simulink model "CaseStudy_Simulink"  (R2019b)
settings: Solver=VariableStepAuto  StartTime=0.0  StopTime=950  RelTol=1e-3
model workspace (MAT data in the model file):
  Making_Order = Simulink.Parameter
  Making_Order.Value = 0
  Making_Order.DataType = 'auto'
  Making_Order.Dimensions = [1 1]
undefined symbols (not defined in the file or in its folder): Clculate_ProccessTime, entity, Faulty_Unit_Identification, genNewOrder, m, n, Packaging
settings Model: PacingRate=1.100000  OrderedModelArguments=off  Creator=faedaa  LastModifiedBy=faedaa

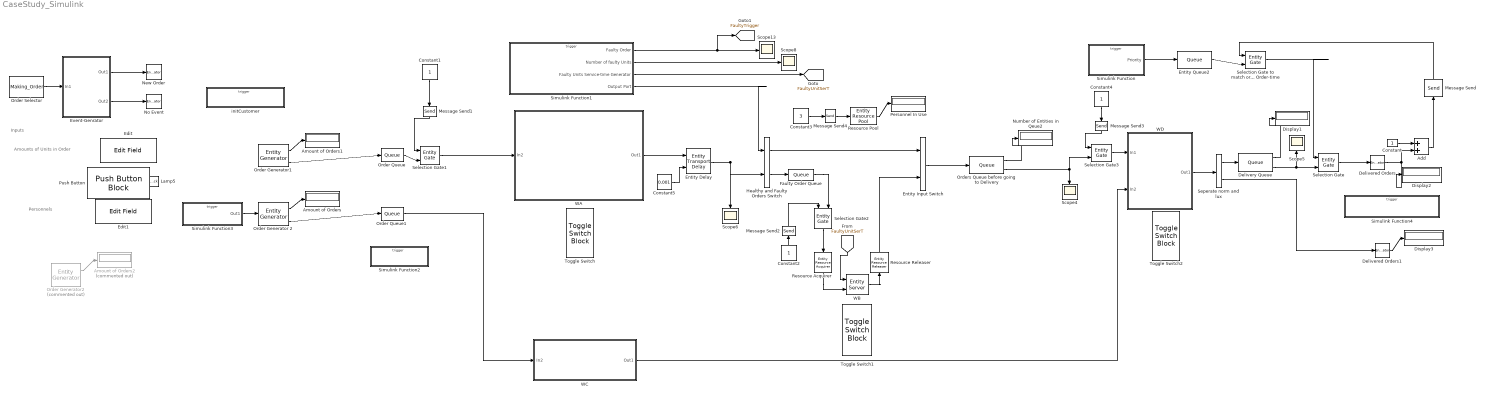
== system CaseStudy_Simulink ==
  note: Inputs
  note: Amounts of Units in Order
  note: Personnels
  Add : Sum  Inputs=2
  Amount of Orders : Display
  Amount of Orders1 : Display
  Amount of Orders2 : Display  Commented=on
  Constant{,1..2,4} (4 alike) : Constant
  Constant3 : Constant  Value=3
  Constant5 : Constant  Value=0.001
  Delivered Orders : EntityTerminator  InputPortMessageModes=m  EntryAction=Clculate_ProccessTime(entity.StartTime,entity.pr,entity.Tag_ManualOrders);  NumberEntitiesArrived=on
      settings: OutputPortMap=o0
  Delivered Orders1 : EntityTerminator  InputPortMessageModes=m  EntryAction=Clculate_ProccessTime(entity.StartTime,entity.pr,entity.Tag_ManualOrders);  NumberEntitiesArrived=on
      settings: OutputPortMap=o0
  Delivery Queue : Queue  InputPortMessageModes=m  OutputPortMessageModes=n,m  Capacity=inf  QueueType=Priority  PrioritySource=pr  NumberEntitiesInBlock=on
      settings: OutputPortMap=o1,o5
  Display1 : Display
  Display2 : Display
  Display3 : Display
  Edit : EditField  LabelPosition=Hide  ShowInitialText=on  Alignment=Center
  Edit1 : EditField  LabelPosition=Hide  ShowInitialText=on  Alignment=Center
  Entity Delay : EntityTransportDelay  InputPortMessageModes=m,n  OutputPortMessageModes=m  Capacity=1
  Entity Input Switch : EntityInputSwitch  InputPortMessageModes=m,m  OutputPortMessageModes=m
  Entity Queue2 : Queue  InputPortMessageModes=m  OutputPortMessageModes=m  Capacity=inf
  Event-Genrator : Subsystem
  Faulty Order Queue : Queue  InputPortMessageModes=m  OutputPortMessageModes=m  Capacity=inf
  Healthy and Faulty Orders Switch : EntityOutputSwitch  InputPortMessageModes=m,m  OutputPortMessageModes=m,m  SwitchingCriterion=From control port  SwitchAttributeName=Attribute1
      settings: InputPortMap=u0,u1
  Lamp5 : LampBlock  LabelPosition=Hide
  Message Send{,1..4} (5 alike) : Send  OutputPortMessageModes=m
  New Order : EntityTerminator  InputPortMessageModes=m  EntryAction=genNewOrder();
  No Event : EntityTerminator  InputPortMessageModes=m
  Number of Entities in Qeue2 : Display
  Order Generator 2 : EntityGenerator  InputPortMessageModes=m  OutputPortMessageModes=n,m  GenerationMethod=Event-based  TimeSource=MATLAB action  IntergenerationTimeAction=|  GenerateAction=entity.Units = Units_Assign();  AttributeName=Units|pr|StartTime|Tag_ManualOrders  AttributeInitialValue=1|0|0|2  NumberEntitiesDeparted=on  EntityType=Structured  EntityTypeName=Entity  DataInitialValue=Units_Amounts
      | persistent rngInit;
      | if isempty(rngInit)
      |     seed = 12345;
      |     rng(seed);
      |     rngInit = true;
      | end
      | 
      | % Pattern: Exponential distribution
      | mu = 30;
      | dt = -mu * log(1 - rand());
      settings: InputPortMap=u0  OutputPortMap=o0,o3
  Order Generator1 : EntityGenerator  OutputPortMessageModes=n,m  TimeSource=MATLAB action  Period=0  IntergenerationTimeAction=|  GenerateAction=|  AttributeName=Units|pr|StartTime|Tag_ManualOrders  AttributeInitialValue=1|0|0|1  NumberEntitiesDeparted=on  EntityType=Structured  EntityTypeName=Entity
      | persistent rngInit;
      | if isempty(rngInit)
      |     seed = 1;
      |     rng(seed);
      |     rngInit = true;
      | end
      | 
      | % Pattern: Exponential distribution
      | mu = 40;
      | dt = -mu * log(1 - rand());
      | persistent rngInit;
      | if isempty(rngInit)
      |     seed = 12345;
      |     rng(seed);
      |     rngInit = true;
      | end
      | 
      | % Pattern: Uniform distribution
      | % m: Minimum, M: Maximum
      | m = 5; M = 100;
      | entity.Units = round(m + (M - m) * rand);
      settings: OutputPortMap=o0,o3
  Order Generator2 : EntityGenerator  Commented=on  OutputPortMessageModes=n,m  TimeSource=MATLAB action  Period=0  IntergenerationTimeAction=|  GenerateEntityAtSimulationStart=off  GenerateAction=|  AttributeName=Units|pr|StartTime|Tag_ManualOrders  AttributeInitialValue=1|0|0|2  NumberEntitiesDeparted=on  EntityType=Structured  EntityTypeName=Entity
      | persistent rngInit;
      | if isempty(rngInit)
      |     seed = 154;
      |     rng(seed);
      |     rngInit = true;
      | end
      | 
      | % Pattern: Exponential distribution
      | mu = 200;
      | dt = -mu * log(1 - rand());
      | persistent rngInit;
      | if isempty(rngInit)
      |     seed = 111;
      |     rng(seed);
      |     rngInit = true;
      | end
      | 
      | % Pattern: Uniform distribution
      | % m: Minimum, M: Maximum
      | m = 1; M = 6;
      | entity.Units = round(m + (M - m) * rand);
      settings: OutputPortMap=o0,o3
  Order Queue : Queue  InputPortMessageModes=m  OutputPortMessageModes=m  Capacity=inf  EntryAction=|
      | persistent idx;
      | if isempty(idx)
      |     idx = 1;
      | end
      | entity.pr = idx
      | idx = idx + 1;
      | 
      | ControlInputpr(entity.pr);
      | 
      | 
      | t = getCurrentTime();
      | entity.StartTime = t/60;
  Order Queue1 : Queue  InputPortMessageModes=m  OutputPortMessageModes=m  Capacity=inf  EntryAction=|
      | persistent id;
      | if isempty(id)
      |     id = 1;
      | end
      | entity.pr = id
      | id = id + 1;
      | 
      | t = getCurrentTime();
      | entity.StartTime = t/60;
  Order Selector : Constant  Value=Making_Order
  Orders Queue before going to Delivery : Queue  InputPortMessageModes=m  OutputPortMessageModes=n,m  Capacity=inf  ExitAction=Packaging(entity.Units)  NumberEntitiesInBlock=on
      settings: OutputPortMap=o1,o5
  Personnel In Use : Display
  Push Button : PushButtonBlock  ButtonText=Make Order
  Resource Acquirer : EntityResourceAcquirer  InputPortMessageModes=m  OutputPortMessageModes=m  ResourceName=WorkerB
      settings: OutputPortMap=o3
  Resource Releaser : EntityResourceReleaser  InputPortMessageModes=m  OutputPortMessageModes=m  ResourceToRelease=Selected  ResourceName=WorkerB  ResourceAmount=1
  Resource Pool : EntityResourcePool  InputPortMessageModes=m  ResourceName=WorkerB  ResourceAmountSource=Change amount through control port  ResourceAmount=2  InitialResourceAmount=0  AmountInUse=on
  Scope{4..6,8,13} (5 alike) : Scope
  Selection Gate : EntityGate  InputPortMessageModes=m,m  OutputPortMessageModes=m  OperatingMode=Selection gate  MatchingAttributeName=pr
  Selection Gate to match orders based on Order-time : EntityGate  InputPortMessageModes=m,m  OutputPortMessageModes=m  OperatingMode=Selection gate  MatchingAttributeName=entity
  Selection Gate1 : EntityGate  InputPortMessageModes=m,m  OutputPortMessageModes=m  MatchingAttributeName=entity
  Selection Gate2 : EntityGate  InputPortMessageModes=m,m  OutputPortMessageModes=m  MatchingAttributeName=entity
  Selection Gate3 : EntityGate  InputPortMessageModes=m,m  OutputPortMessageModes=m  MatchingAttributeName=entity
  "Seperate norm and lux " : EntityOutputSwitch  InputPortMessageModes=m  OutputPortMessageModes=m,m  SwitchingCriterion=From attribute  SwitchAttributeName=Tag_ManualOrders
  Simulink Function : Subsystem  TreatAsAtomicUnit=on
  Simulink Function1 : Subsystem  TreatAsAtomicUnit=on
  Simulink Function2 : Subsystem  TreatAsAtomicUnit=on
  Simulink Function3 : Subsystem  TreatAsAtomicUnit=on
  Simulink Function4 : Subsystem  TreatAsAtomicUnit=on
  Toggle Switch : ToggleSwitchBlock  LabelPosition=Hide
      settings: Values={{'Off', 'On'}, [0 1]}
  Toggle Switch1 : ToggleSwitchBlock  LabelPosition=Hide
      settings: Values={{'Off', 'On'}, [0 1]}
  Toggle Switch2 : ToggleSwitchBlock  LabelPosition=Hide
      settings: Values={{'Off', 'On'}, [0 1]}
  WA : Subsystem
  WB : EntityServer  InputPortMessageModes=n,m  OutputPortMessageModes=m  Capacity=1  ServiceTimeSource=Signal port  ServiceTimeAction=|
      | persistent rngInit;
      | if isempty(rngInit)
      |     seed = 12345;
      |     rng(seed);
      |     rngInit = true;
      | end
      | 
      | % Pattern: Exponential distribution
      | mu = 20;
      | dt = -mu * log(1 - rand());
      settings: InputPortMap=u0,u2
  WC : Subsystem
  WD : Subsystem
  initCustomer : Subsystem  TreatAsAtomicUnit=on
  tag scope: FaultyTrigger=global, FaultyUnitSerT=global
  wires:
  Simulink Function/1(Priority) -> Entity Queue2/1
  Resource Releaser/1 -> Entity Input Switch/2
  Simulink Function1/4(Output Port) -> Healthy and Faulty Orders Switch/1
  Resource Acquirer/1 -> WB/2
  Simulink Function1/2(Number of faulty Units) -> Scope8/1
  Constant/1 -> Add/1
  Entity Queue2/1 -> Selection Gate to match orders based on Order-time/2
  Order Generator 2/1 -> Amount of Orders/1
  Event-Genrator/1(Out1) -> New Order/1
  Orders Queue before going to Delivery/1 -> Number of Entities in Qeue2/1
  Simulink Function1/3(Faulty Units Service-time Generator) -> [FaultyUnitSerT]
  WB/1 -> Resource Releaser/1
  Simulink Function3/1(Out1) -> Order Generator 2/1
  Event-Genrator/2(Out2) -> No Event/1
  Delivery Queue/1 -> Display1/1
  Healthy and Faulty Orders Switch/1 -> Entity Input Switch/1
  Delivery Queue/2 -> Selection Gate/2, Scope5/1
  Order Selector/1 -> Event-Genrator/1(In1)
  Message Send/1 -> Selection Gate to match orders based on Order-time/1
  [FaultyUnitSerT] -> WB/1
  Selection Gate to match orders based on Order-time/1 -> Selection Gate/1
  Add/1 -> Message Send/1
  Healthy and Faulty Orders Switch/2 -> Faulty Order Queue/1
  Delivered Orders/1 -> Add/2, Display2/1
  Simulink Function1/1(Faulty Order) -> Scope13/1, [FaultyTrigger]
  Order Generator1/1 -> Amount of Orders1/1
  Constant1/1 -> Message Send1/1
  Message Send1/1 -> Selection Gate1/1
  Selection Gate1/1 -> WA/1(In2)
  Faulty Order Queue/1 -> Selection Gate2/2
  Selection Gate2/1 -> Resource Acquirer/1
  Constant2/1 -> Message Send2/1
  Message Send2/1 -> Selection Gate2/1
  Constant4/1 -> Message Send3/1
  Message Send3/1 -> Selection Gate3/1
  Orders Queue before going to Delivery/2 -> Selection Gate3/2, Scope4/1
  Selection Gate3/1 -> WD/1(In1)
  Constant3/1 -> Message Send4/1
  Message Send4/1 -> Resource Pool/1
  Resource Pool/1 -> Personnel In Use/1
  Constant5/1 -> Entity Delay/2
  WA/1(Out1) -> Entity Delay/1
  Entity Delay/1 -> Scope6/1, Healthy and Faulty Orders Switch/2
  Order Generator1/2 -> Order Queue/1
  WC/1(Out1) -> WD/2(In2)
  Entity Input Switch/1 -> Orders Queue before going to Delivery/1
  Order Queue/1 -> Selection Gate1/2
  Order Queue1/1 -> WC/1(In2)
  WD/1(Out1) -> "Seperate norm and lux "/1
  "Seperate norm and lux "/1 -> Delivery Queue/1
  "Seperate norm and lux "/2 -> Delivered Orders1/1
  Delivered Orders1/1 -> Display3/1
  Selection Gate/1 -> Delivered Orders/1
  Order Generator2/1 -> Amount of Orders2/1
  Order Generator 2/2 -> Order Queue1/1

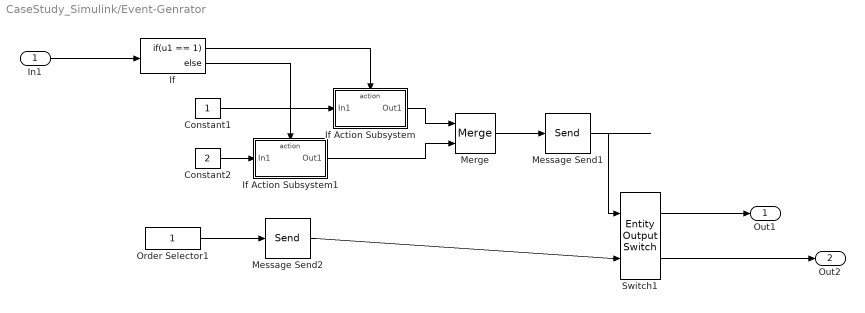
== system CaseStudy_Simulink/Event-Genrator ==
  In1 : Inport
  Constant1 : Constant
  Constant2 : Constant  Value=2
  If : If  IfExpression=u1 == 1
  If Action Subsystem : Subsystem  TreatAsAtomicUnit=on
  If Action Subsystem1 : Subsystem  TreatAsAtomicUnit=on
  Merge : Merge
  Message Send1 : Send  OutputPortMessageModes=m
  Message Send2 : Send  OutputPortMessageModes=m
  Order Selector1 : Constant
  Switch1 : EntityOutputSwitch  InputPortMessageModes=m,m  OutputPortMessageModes=m,m  SwitchingCriterion=From control port  SwitchAttributeName=Attribute1  InitialPortSelection=2
      settings: InputPortMap=u0,u1
  Out1 : Outport
  Out2 : Outport  Port=2
  wires:
  If Action Subsystem/1(Out1) -> Merge/1
  Message Send1/1 -> Switch1/1
  Switch1/2 -> Out2/1
  Constant2/1 -> If Action Subsystem1/1(In1)
  Constant1/1 -> If Action Subsystem/1(In1)
  If/2 -> If Action Subsystem1/Action
  If/1 -> If Action Subsystem/Action
  Message Send2/1 -> Switch1/2
  If Action Subsystem1/1(Out1) -> Merge/2
  Order Selector1/1 -> Message Send2/1
  Merge/1 -> Message Send1/1
  In1/1 -> If/1
  Switch1/1 -> Out1/1

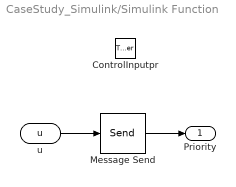
== system CaseStudy_Simulink/Simulink Function ==
  ControlInputpr : TriggerPort  TriggerType=function-call  IsSimulinkFunction=on  FunctionName=ControlInputpr  VariantControl=(inherit)
  Message Send : Send  OutputPortMessageModes=m
  u : ArgIn  DisableCoverage=on  ArgumentName=u
  Priority : Outport
  wires:
  Message Send/1 -> Priority/1
  u/1 -> Message Send/1

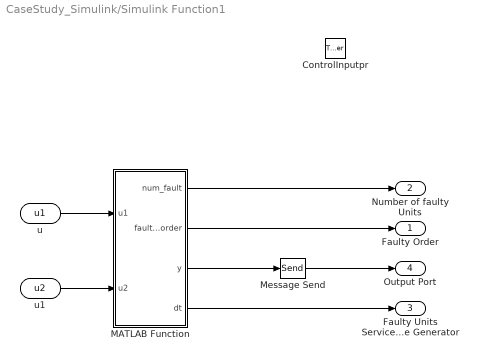
== system CaseStudy_Simulink/Simulink Function1 ==
  ControlInputpr : TriggerPort  TriggerType=function-call  IsSimulinkFunction=on  FunctionName=Faulty_Unit_Identification  VariantControl=(inherit)
  MATLAB Function : MATLAB Function  TreatAsAtomicUnit=on
  Message Send : Send  OutputPortMessageModes=m
  u : ArgIn  DisableCoverage=on  ArgumentName=u1
  u1 : ArgIn  DisableCoverage=on  Port=2  ArgumentName=u2
  Faulty Order : Outport
  Number of faulty Units : Outport  Port=2
  Faulty Units Service-time Generator : Outport  Port=3
  Output Port : Outport  Port=4
  wires:
  Message Send/1 -> Output Port/1
  u/1 -> MATLAB Function/1(u1)
  MATLAB Function/3(y) -> Message Send/1
  MATLAB Function/4(dt) -> Faulty Units Service-time Generator/1
  u1/1 -> MATLAB Function/2(u2)
  MATLAB Function/1(num_fault) -> Number of faulty Units/1
  MATLAB Function/2(faulty_order) -> Faulty Order/1

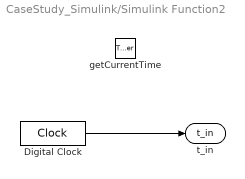
== system CaseStudy_Simulink/Simulink Function2 ==
  getCurrentTime : TriggerPort  TriggerType=function-call  IsSimulinkFunction=on  FunctionName=getCurrentTime  VariantControl=Variant
  Digital Clock : DigitalClock  SampleTime=-1
  t_in : ArgOut  DisableCoverage=on  ArgumentName=t_in
  wires:
  Digital Clock/1 -> t_in/1

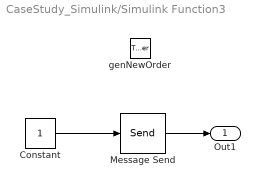
== system CaseStudy_Simulink/Simulink Function3 ==
  genNewOrder : TriggerPort  TriggerType=function-call  IsSimulinkFunction=on  FunctionName=genNewOrder  VariantControl=Variant
  Constant : Constant
  Message Send : Send  OutputPortMessageModes=m
  Out1 : Outport  VectorParamsAs1DForOutWhenUnconnected=off
  wires:
  Constant/1 -> Message Send/1
  Message Send/1 -> Out1/1

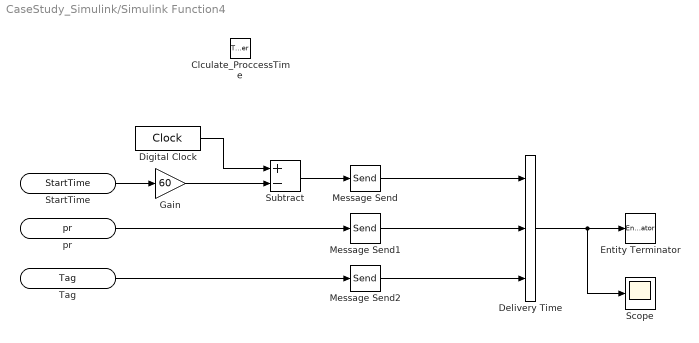
== system CaseStudy_Simulink/Simulink Function4 ==
  Clculate_ProccessTime : TriggerPort  TriggerType=function-call  IsSimulinkFunction=on  FunctionName=Clculate_ProccessTime  VariantControl=Variant
  "Delivery Time " : EntityInputSwitch  InputPortMessageModes=m,m,m  OutputPortMessageModes=m  NumberInputPorts=3
      settings: InputPortMap=u1,u2,u3
  Digital Clock : DigitalClock  SampleTime=-1
  Entity Terminator : EntityTerminator  InputPortMessageModes=m
  Gain : Gain  Gain=60
  Message Send : Send  OutputPortMessageModes=m
  Message Send1 : Send  OutputPortMessageModes=m
  Message Send2 : Send  OutputPortMessageModes=m
  Scope : Scope
  Subtract : Sum  Inputs=+-
  StartTime : ArgIn  DisableCoverage=on  ArgumentName=StartTime
  pr : ArgIn  DisableCoverage=on  Port=2  ArgumentName=pr
  Tag : ArgIn  DisableCoverage=on  Port=3  ArgumentName=Tag
  wires:
  StartTime/1 -> Gain/1
  Digital Clock/1 -> Subtract/1
  Subtract/1 -> Message Send/1
  pr/1 -> Message Send1/1
  "Delivery Time "/1 -> Scope/1, Entity Terminator/1
  Message Send/1 -> "Delivery Time "/1
  Message Send1/1 -> "Delivery Time "/2
  Gain/1 -> Subtract/2
  Tag/1 -> Message Send2/1
  Message Send2/1 -> "Delivery Time "/3

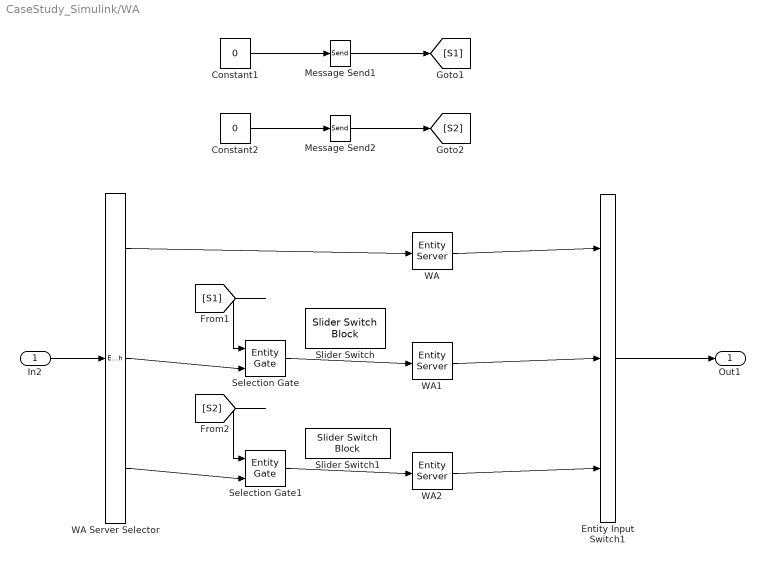
== system CaseStudy_Simulink/WA ==
  In2 : Inport
  Constant1 : Constant  Value=0
  Constant2 : Constant  Value=0
  Entity Input Switch1 : EntityInputSwitch  InputPortMessageModes=m,m,m  OutputPortMessageModes=m  NumberInputPorts=3
      settings: InputPortMap=u1,u2,u3
  Message Send1 : Send  OutputPortMessageModes=m
  Message Send2 : Send  OutputPortMessageModes=m
  Selection Gate : EntityGate  InputPortMessageModes=m,m  OutputPortMessageModes=m  MatchingAttributeName=entity
  Selection Gate1 : EntityGate  InputPortMessageModes=m,m  OutputPortMessageModes=m  MatchingAttributeName=entity
  Slider Switch : SliderSwitchBlock  LabelPosition=Hide
      settings: Values={{'Off', 'On'}, [0 1]}
  Slider Switch1 : SliderSwitchBlock  LabelPosition=Hide
      settings: Values={{'Off', 'On'}, [0 1]}
  WA : EntityServer  InputPortMessageModes=m  OutputPortMessageModes=m  Capacity=2  ServiceTimeSource=MATLAB action  ServiceTimeAction=|  ExitAction=Faulty_Unit_Identification(entity.Units,entity.pr);
      | persistent rngInit;
      | if isempty(rngInit)
      |     seed = 12;
      |     rng(seed);
      |     rngInit = true;
      | end
      | 
      | % Pattern: Exponential distribution
      | mu = 0.5;
      | 
      | Ed_perU = zeros(entity.Units,1);
      | for j=1:entity.Units
      |     Ed_perU(j) = -mu * log(1 - rand());
      | end
      | 
      | dt = sum(Ed_perU);
  WA Server Selector : EntityOutputSwitch  InputPortMessageModes=m  OutputPortMessageModes=m,m,m  NumberOutputPorts=3  SwitchAttributeName=Attribute1
      settings: OutputPortMap=o0,o1,o2
  WA1 : EntityServer  InputPortMessageModes=m  OutputPortMessageModes=m  Capacity=1  ServiceTimeSource=MATLAB action  ServiceTimeAction=|  ExitAction=Faulty_Unit_Identification(entity.Units,entity.pr);
      | persistent rngInit;
      | if isempty(rngInit)
      |     seed = 123;
      |     rng(seed);
      |     rngInit = true;
      | end
      | 
      | % Pattern: Exponential distribution
      | mu = 1;
      | 
      | Ed_perU = zeros(entity.Units,1);
      | for j=1:entity.Units
      |     Ed_perU(j) = -mu * log(1 - rand());
      | end
      | 
      | dt = sum(Ed_perU);
  WA2 : EntityServer  InputPortMessageModes=m  OutputPortMessageModes=m  Capacity=1  ServiceTimeSource=MATLAB action  ServiceTimeAction=|  ExitAction=Faulty_Unit_Identification(entity.Units,entity.pr);
      | persistent rngInit;
      | if isempty(rngInit)
      |     seed = 12345;
      |     rng(seed);
      |     rngInit = true;
      | end
      | 
      | % Pattern: Exponential distribution
      | mu = 1;
      | 
      | Ed_perU = zeros(entity.Units,1);
      | for j=1:entity.Units
      |     Ed_perU(j) = -mu * log(1 - rand());
      | end
      | 
      | dt = sum(Ed_perU);
  Out1 : Outport
  wires:
  WA Server Selector/2 -> Selection Gate/2
  [S2] -> Selection Gate1/1
  WA2/1 -> Entity Input Switch1/3
  WA Server Selector/3 -> Selection Gate1/2
  WA1/1 -> Entity Input Switch1/2
  Selection Gate/1 -> WA1/1
  Selection Gate1/1 -> WA2/1
  WA/1 -> Entity Input Switch1/1
  [S1] -> Selection Gate/1
  Entity Input Switch1/1 -> Out1/1
  Constant1/1 -> Message Send1/1
  Message Send2/1 -> [S2]
  Constant2/1 -> Message Send2/1
  Message Send1/1 -> [S1]
  In2/1 -> WA Server Selector/1
  WA Server Selector/1 -> WA/1

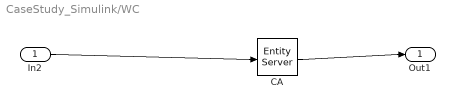
== system CaseStudy_Simulink/WC ==
  In2 : Inport
  CA : EntityServer  InputPortMessageModes=m  OutputPortMessageModes=m  Capacity=1  ServiceTimeSource=MATLAB action  ServiceTimeAction=|
      | persistent rngInit;
      | if isempty(rngInit)
      |     seed = 23;
      |     rng(seed);
      |     rngInit = true;
      | end
      | 
      | % Pattern: Exponential distribution
      | mu = 8;
      | 
      | Ed_perU = zeros(entity.Units,1);
      | for j=1:entity.Units
      |     Ed_perU(j) = -mu * log(1 - rand());
      | end
      | 
      | dt = sum(Ed_perU);
  Out1 : Outport
  wires:
  CA/1 -> Out1/1
  In2/1 -> CA/1

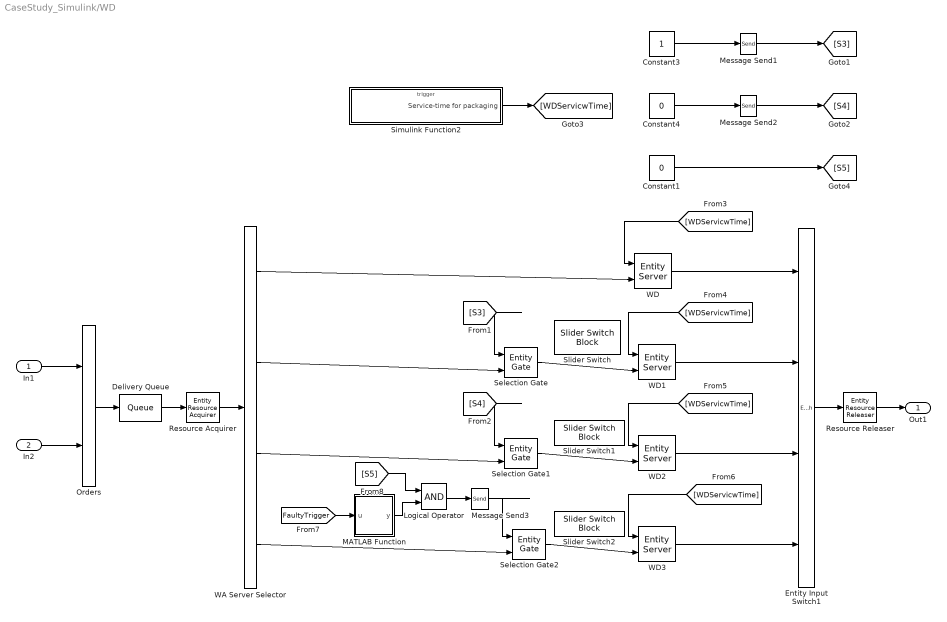
== system CaseStudy_Simulink/WD ==
  In1 : Inport
  In2 : Inport  Port=2
  Constant1 : Constant  Value=0
  Constant3 : Constant
  Constant4 : Constant  Value=0
  Delivery Queue : Queue  InputPortMessageModes=m  OutputPortMessageModes=m  Capacity=inf  QueueType=Priority  PrioritySource=Tag_ManualOrders  SortingDirection=Descending
  Entity Input Switch1 : EntityInputSwitch  InputPortMessageModes=m,m,m,m  OutputPortMessageModes=m  NumberInputPorts=4
      settings: InputPortMap=u1,u2,u3,u4
  Logical Operator : Logic  AllPortsSameDT=off  OutDataTypeStr=boolean
  MATLAB Function : MATLAB Function  TreatAsAtomicUnit=on
  Message Send1 : Send  OutputPortMessageModes=m
  Message Send2 : Send  OutputPortMessageModes=m
  Message Send3 : Send  OutputPortMessageModes=m
  Orders : EntityInputSwitch  InputPortMessageModes=m,m  OutputPortMessageModes=m
  Resource Acquirer : EntityResourceAcquirer  InputPortMessageModes=m  OutputPortMessageModes=m  ResourceName=WorkerB
      settings: OutputPortMap=o3
  Resource Releaser : EntityResourceReleaser  InputPortMessageModes=m  OutputPortMessageModes=m  ResourceToRelease=Selected  ResourceName=WorkerB  ResourceAmount=1
  Selection Gate : EntityGate  InputPortMessageModes=m,m  OutputPortMessageModes=m  MatchingAttributeName=entity
  Selection Gate1 : EntityGate  InputPortMessageModes=m,m  OutputPortMessageModes=m  MatchingAttributeName=entity
  Selection Gate2 : EntityGate  InputPortMessageModes=m,m  OutputPortMessageModes=m  MatchingAttributeName=entity
  Simulink Function2 : Subsystem  TreatAsAtomicUnit=on
  Slider Switch : SliderSwitchBlock  LabelPosition=Hide
      settings: Values={{'Off', 'On'}, [0 1]}
  Slider Switch1 : SliderSwitchBlock  LabelPosition=Hide
      settings: Values={{'Off', 'On'}, [0 1]}
  Slider Switch2 : SliderSwitchBlock  LabelPosition=Hide
      settings: Values={{'Off', 'On'}, [0 1]}
  WA Server Selector : EntityOutputSwitch  InputPortMessageModes=m  OutputPortMessageModes=m,m,m,m  NumberOutputPorts=4  SwitchAttributeName=Attribute1
      settings: OutputPortMap=o0,o1,o2,o3
  WD : EntityServer  InputPortMessageModes=n,m  OutputPortMessageModes=m  Capacity=1  ServiceTimeSource=Signal port  ServiceTimeAction=|
      | persistent rngInit;
      | if isempty(rngInit)
      |     seed = 12345;
      |     rng(seed);
      |     rngInit = true;
      | end
      | 
      | % Pattern: Exponential distribution
      | mu = 30;
      | dt = -mu * log(1 - rand());
      settings: InputPortMap=u0,u2
  WD1 : EntityServer  InputPortMessageModes=n,m  OutputPortMessageModes=m  Capacity=1  ServiceTimeSource=Signal port  ServiceTimeAction=|
      | persistent rngInit;
      | if isempty(rngInit)
      |     seed = 12345;
      |     rng(seed);
      |     rngInit = true;
      | end
      | 
      | % Pattern: Exponential distribution
      | mu = 30;
      | dt = -mu * log(1 - rand());
      settings: InputPortMap=u0,u2
  WD2 : EntityServer  InputPortMessageModes=n,m  OutputPortMessageModes=m  Capacity=1  ServiceTimeSource=Signal port  ServiceTimeAction=|
      | persistent rngInit;
      | if isempty(rngInit)
      |     seed = 12345;
      |     rng(seed);
      |     rngInit = true;
      | end
      | 
      | % Pattern: Exponential distribution
      | mu = 30;
      | dt = -mu * log(1 - rand());
      settings: InputPortMap=u0,u2
  WD3 : EntityServer  InputPortMessageModes=n,m  OutputPortMessageModes=m  Capacity=1  ServiceTimeSource=Signal port  ServiceTimeAction=|
      | persistent rngInit;
      | if isempty(rngInit)
      |     seed = 12345;
      |     rng(seed);
      |     rngInit = true;
      | end
      | 
      | % Pattern: Exponential distribution
      | mu = 30;
      | dt = -mu * log(1 - rand());
      settings: InputPortMap=u0,u2
  Out1 : Outport
  wires:
  Message Send1/1 -> [S3]
  Constant4/1 -> Message Send2/1
  Message Send2/1 -> [S4]
  Constant3/1 -> Message Send1/1
  Entity Input Switch1/1 -> Resource Releaser/1
  [S3] -> Selection Gate/1
  WA Server Selector/1 -> WD/2
  WD/1 -> Entity Input Switch1/1
  Selection Gate1/1 -> WD2/2
  Selection Gate/1 -> WD1/2
  WD1/1 -> Entity Input Switch1/2
  WA Server Selector/3 -> Selection Gate1/2
  WD2/1 -> Entity Input Switch1/3
  [S4] -> Selection Gate1/1
  WA Server Selector/2 -> Selection Gate/2
  Simulink Function2/1(Service-time for packaging) -> [WDServicwTime]
  [WDServicwTime] -> WD/1
  [WDServicwTime] -> WD1/1
  [WDServicwTime] -> WD2/1
  [WDServicwTime] -> WD3/1
  WA Server Selector/4 -> Selection Gate2/2
  [FaultyTrigger] -> MATLAB Function/1(u)
  Message Send3/1 -> Selection Gate2/1
  Selection Gate2/1 -> WD3/2
  WD3/1 -> Entity Input Switch1/4
  Resource Acquirer/1 -> WA Server Selector/1
  Resource Releaser/1 -> Out1/1
  Constant1/1 -> [S5]
  Logical Operator/1 -> Message Send3/1
  MATLAB Function/1(y) -> Logical Operator/2
  [S5] -> Logical Operator/1
  In1/1 -> Orders/1
  In2/1 -> Orders/2
  Orders/1 -> Delivery Queue/1
  Delivery Queue/1 -> Resource Acquirer/1

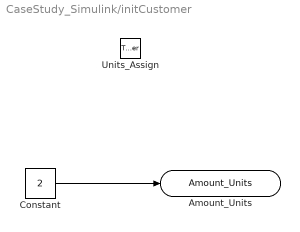
== system CaseStudy_Simulink/initCustomer ==
  Units_Assign : TriggerPort  TriggerType=function-call  IsSimulinkFunction=on  FunctionName=Units_Assign  VariantControl=Variant
  Constant : Constant  Value=2
  Amount_Units : ArgOut  ArgumentName=Amount_Units
  wires:
  Constant/1 -> Amount_Units/1

== system CaseStudy_Simulink/Event-Genrator/If Action Subsystem ==
  In1 : Inport
  Action Port : ActionPort  ActionPortLabel=if(u1 == 1)
  Out1 : Outport
  wires:
  In1/1 -> Out1/1

== system CaseStudy_Simulink/Event-Genrator/If Action Subsystem1 ==
  In1 : Inport
  Action Port : ActionPort  ActionPortLabel=else
  Out1 : Outport
  wires:
  In1/1 -> Out1/1

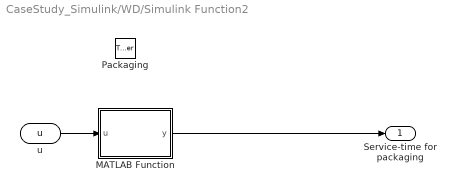
== system CaseStudy_Simulink/WD/Simulink Function2 ==
  Packaging : TriggerPort  TriggerType=function-call  IsSimulinkFunction=on  FunctionName=Packaging  VariantControl=(inherit)
  MATLAB Function : MATLAB Function  TreatAsAtomicUnit=on
  u : ArgIn  DisableCoverage=on  ArgumentName=u
  Service-time for packaging : Outport
  wires:
  MATLAB Function/1(y) -> Service-time for packaging/1
  u/1 -> MATLAB Function/1(u)

== matlab function CaseStudy_Simulink/WD/Simulink Function2/MATLAB Function ==
  data: u input; y output
function y = fcn(u)
persistent rnginit2
if isempty(rnginit2)
    seed = 1819;
    rng(seed);
    rnginit2 = true;
end

p = u/30;
num = ceil(p);
mu = 24;
y = -mu * log(1 - rand()) * num;

== matlab function CaseStudy_Simulink/Simulink Function1/MATLAB Function ==
  data: num_fault output; faulty_order output; u1 input; y output; dt output; u2 input
function [num_fault,faulty_order,y, dt] = fcn(u1,u2)

persistent rnginit1
if isempty(rnginit1)
    seed = 1818;
    rng(seed);
    rnginit1 = true;
end
y = 1;
num_fault = 0;
faulty_order = 0;
mu = 6;
p = rand(u1,1);

for i=1:u1
    
    if p(i)<0.01
        y = 2;
        num_fault = num_fault + 1;
        faulty_order = u2;
    end
    
end

if num_fault>0
    x = zeros(num_fault,1);
    for j=1:num_fault
        x(j) = -mu * log(1 - rand());
    end
    dt = sum(x);
else
    dt = 0;
end

== matlab function CaseStudy_Simulink/WD/MATLAB Function ==
  data: u input; y output
function y = fcn(u)

if u==0
    y = 1;
else
    y = 0;
end
